simulink model "modulation_example_ofdm"  (R2015b)
settings: Solver=VariableStepAuto  StartTime=0.0  StopTime=1  RelTol=1e-3
libraries: commdigbbndpm3 x2, commofdm x2, commseqgen3 x1
settings Model: Creator=liujj-d  LastModifiedBy=liujj-d

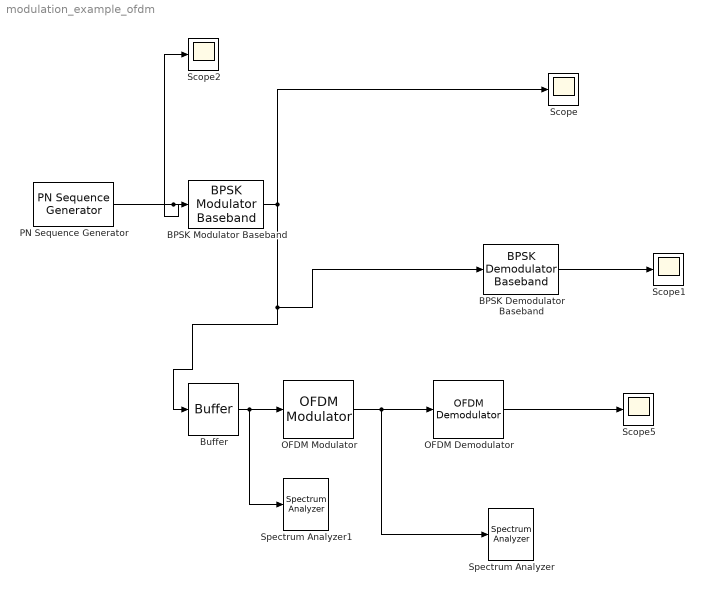
== system modulation_example_ofdm ==
  BPSK Demodulator Baseband : commdigbbndpm3/BPSK Demodulator Baseband  Ph=0  DecType=Hard decision  VarSource=Dialog  Variance=1  outDtype=Inherit via internal rule  derotateFactorWordLen=16
  BPSK Modulator Baseband : commdigbbndpm3/BPSK Modulator Baseband  Ph=0  outDtype=double  outWordLen=16  outUDDataType=sfix(16)  outFracLenMode=Best precision  outFracLen=15
  Buffer : Buffer  N=52  TreatMby1Signals=One channel  OutputFrames=off
  OFDM Demodulator : commofdm/OFDM Demodulator  FFTLength=64  NumGuardBandCarriers=[6; 5]  RemoveDCCarrier=off  PilotOutputPort=off  PilotCarrierIndices=[12; 26; 40; 54]  CyclicPrefixLength=16  NumSymbols=1  NumReceiveAntennas=1  SimulateUsing=Interpreted execution
  OFDM Modulator : commofdm/OFDM Modulator  FFTLength=64  NumGuardBandCarriers=[6; 5]  InsertDCNull=on  PilotInputPort=off  PilotCarrierIndices=[12; 26; 40; 54]  CyclicPrefixLength=16  Windowing=off  WindowLength=1  NumSymbols=1  NumTransmitAntennas=1  SimulateUsing=Interpreted execution
  PN Sequence Generator : commseqgen3/PN Sequence Generator  poly='z^6 + z + 1'  ini_sta=[0 0 0 0 0 1]  outBitMaskSource=Dialog parameter  shift=0  outVarSiz=off  maxOutSizeMode=Dialog parameter  maxOutSize=[10 1]  Ts=0.0001  sampPerFrame=1  reset=off  bitPackedOutputs=off  outDataType=double  numPackedBits=8  bitPackDataSigned=off  bitPackedOutDType=double
  Scope{,1..2,5} (4 alike) : Scope
  Spectrum Analyzer : SpectrumAnalyzer
  Spectrum Analyzer1 : SpectrumAnalyzer
  wires:
  PN Sequence Generator/1 -> Scope2/1, BPSK Modulator Baseband/1
  BPSK Modulator Baseband/1 -> Buffer/1, BPSK Demodulator Baseband/1, Scope/1
  BPSK Demodulator Baseband/1 -> Scope1/1
  OFDM Modulator/1 -> Spectrum Analyzer/1, OFDM Demodulator/1
  OFDM Demodulator/1 -> Scope5/1
  Buffer/1 -> Spectrum Analyzer1/1, OFDM Modulator/1
